simulink model "TemplateNoLineal"  (R2018a)
settings: Solver=ode45  StartTime=0.0  StopTime=10  FixedStep=0.001  RelTol=1e-3
undefined symbols (not defined in the file or in its folder): Gss, K, ki, L, uo, xo, yo
settings Model: Creator=aghersin  LastModifiedBy=aghersin

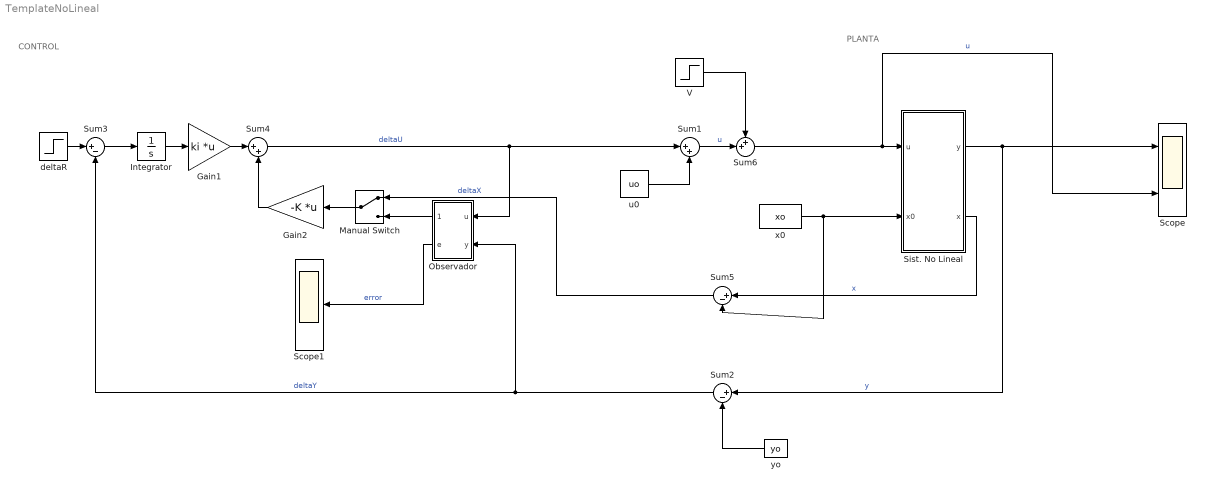
== system TemplateNoLineal ==
  note: CONTROL
  note: PLANTA
  Gain1 : Gain  Gain=ki  Multiplication=Matrix(K*u)
  Gain2 : Gain  Gain=-K  Multiplication=Matrix(K*u)
  Integrator : Integrator
  Manual Switch : ManualSwitch
  Observador : Subsystem
  Scope : Scope  NumInputPorts=2
  Scope1 : Scope
  "Sist. No Lineal " : Subsystem
  Sum1 : Sum  Inputs=|++
  Sum2 : Sum  Inputs=|+-
  Sum3 : Sum  Inputs=|+-
  Sum4 : Sum  Inputs=|++
  Sum5 : Sum  Inputs=|+-
  Sum6 : Sum  Inputs=++|
  V : Step  Time=5  After=3  SampleTime=0
  deltaR : Step  Time=.1  After=0.1  SampleTime=0
  u0 : Constant  Value=uo
  x0 : Constant  Value=xo
  yo : Constant  Value=yo
  wires:
  Gain2/1 -> Sum4/2
  Sum4/1 -> Sum1/1, Observador/1(u)  "deltaU"
  deltaR/1 -> Sum3/1
  Sum3/1 -> Integrator/1
  u0/1 -> Sum1/2
  Integrator/1 -> Gain1/1
  Sum1/1 -> Sum6/2  "u"
  Observador/2(e) -> Scope1/1  "error"
  Manual Switch/1 -> Gain2/1
  Observador/1(xhat) -> Manual Switch/2
  Gain1/1 -> Sum4/1
  V/1 -> Sum6/1
  Sum6/1 -> Scope/2, "Sist. No Lineal "/1(u)  "u"
  "Sist. No Lineal "/2(x) -> Sum5/1  "x"
  "Sist. No Lineal "/1(y) -> Scope/1, Sum2/1  "y"
  x0/1 -> Sum5/2, "Sist. No Lineal "/2(x0)
  yo/1 -> Sum2/2
  Sum2/1 -> Observador/2(y), Sum3/2  "deltaY"
  Sum5/1 -> Manual Switch/1  "deltaX"

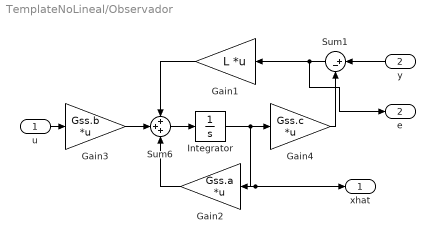
== system TemplateNoLineal/Observador ==
  u : Inport
  y : Inport  Port=2
  Gain1 : Gain  Gain=L  Multiplication=Matrix(K*u)
  Gain2 : Gain  Gain=Gss.a  Multiplication=Matrix(K*u)
  Gain3 : Gain  Gain=Gss.b  Multiplication=Matrix(K*u)
  Gain4 : Gain  Gain=Gss.c  Multiplication=Matrix(K*u)
  Integrator : Integrator
  Sum1 : Sum  Inputs=|+-
  Sum6 : Sum  Inputs=+++
  xhat : Outport
  e : Outport  Port=2
  wires:
  Gain2/1 -> Sum6/3
  Integrator/1 -> Gain4/1, xhat/1, Gain2/1
  u/1 -> Gain3/1
  Sum6/1 -> Integrator/1
  Gain4/1 -> Sum1/2
  Gain3/1 -> Sum6/2
  Sum1/1 -> e/1, Gain1/1
  y/1 -> Sum1/1
  Gain1/1 -> Sum6/1

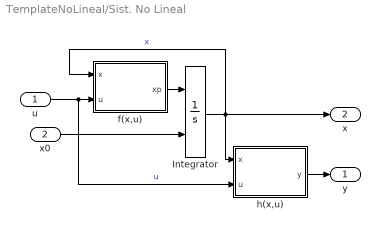
== system TemplateNoLineal/Sist. No Lineal  ==
  u : Inport
  x0 : Inport  Port=2
  Integrator : Integrator  InitialConditionSource=external
  f(x,u) : MATLAB Function  TreatAsAtomicUnit=on
  h(x,u) : MATLAB Function  TreatAsAtomicUnit=on
  y : Outport
  x : Outport  Port=2
  wires:
  h(x,u)/1(y) -> y/1
  u/1 -> h(x,u)/2(u), f(x,u)/2(u)  "u"
  f(x,u)/1(xp) -> Integrator/1
  Integrator/1 -> h(x,u)/1(x), x/1, f(x,u)/1(x)  "x"
  x0/1 -> Integrator/2

== matlab function TemplateNoLineal/Sist. No Lineal /f(x,u) ==
  data: x input; u input; xp output
function xp = f(x,u)

xp1=-sqrt(x(1)-x(2))+u;
xp2=sqrt(x(1)-x(2))+sqrt(x(2));

xp=[xp1;xp2];

== matlab function TemplateNoLineal/Sist. No Lineal /h(x,u) ==
  data: x input; u input; y output
function y = h(x,u)

y=x(1);
